simulink model "Homework1"  (R2015b)
settings: Solver=VariableStepAuto  StartTime=1  StopTime=2  RelTol=1e-3
settings Model: Creator=YagfarovRauf  LastModifiedBy=YagfarovRauf

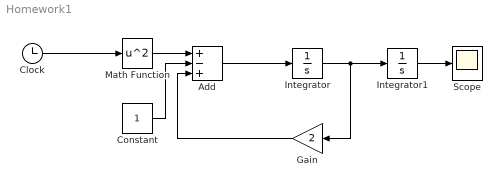
== system Homework1 ==
  Add : Sum  Inputs=+-+
  Clock : Clock
  Constant : Constant
  Gain : Gain  Gain=2
  Integrator : Integrator  InitialCondition=-3/4
  Integrator1 : Integrator  InitialCondition=-1/6
  Math Function : Math  Operator=square  SaturateOnIntegerOverflow=on
  Scope : Scope
  wires:
  Integrator/1 -> Gain/1, Integrator1/1
  Add/1 -> Integrator/1
  Gain/1 -> Add/3
  Constant/1 -> Add/2
  Integrator1/1 -> Scope/1
  Math Function/1 -> Add/1
  Clock/1 -> Math Function/1
